simulink library "sixDoFDynamicsCoupled"  (R2020a)
settings: Solver=VariableStepAuto  StartTime=0.0  StopTime=10.0  RelTol=1e-3
undefined symbols (not defined in the file): initPos, vcl
libraries: vrlib x7, eulAng2RotMat_ul x1, eulDot x1
settings Model: Creator=jldanie5  LastModifiedBy=Ayaz
settings DataIOCC: ReturnWorkspaceOutputs=off
settings DebuggingCC: ArithmeticOperatorsInVariantConditions=warning
settings SFSimCC: CustomCodeUndefinedFunction=UseInterfaceOnly

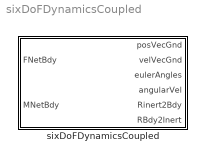
== system sixDoFDynamicsCoupled ==
  sixDoFDynamicsCoupled : Subsystem  VariantControl=(default)  mask{massMatrix=vcl.M6x6.Value, addedMassMatrix=vcl.Ma6x6.Value, rCM_LE=vcl.rCM_B.Value, initPosCM=vcl.initPosVecGnd.Value, initVelCM=vcl.initVelVecBdy.Value, initEulAngs=vcl.initEulAng.Value, initAngVel=vcl.initAngVelVec.Value}
      mask prompts: massMatrix "6x6 Mass Matrix"; addedMassMatrix "6x6 Added Mass Matrix"; rCM_LE "Center of mass position vec wrt leading edge in body frame"; initPosCM "Initial position"; initVelCM "Initial velocity"; initEulAngs "Initial Euler Angles"; initAngVel "Initial Angular Velocity Vec"
      mask init:
      | Mnet = massMatrix - addedMassMatrix;
      | invMnet = inv(Mnet);
      | mAddedTimesMInvMinusEye = addedMassMatrix*inv(massMatrix) - eye(6);
      | 
      | % mass
      | m = massMatrix(1,1);
      | % inertia about body frame origin
      | J = massMatrix(4:6,4:6);
      | % initial velocity of body frame origin
      | initVelB = initVelCM - cross(initAngVel,rCM_LE);
      mask DialogControl Container6 Prompt: Mass Matrices
      mask DialogControl Container4 Prompt: Point Locations
      mask DialogControl Container3 Prompt: Initial Conditions

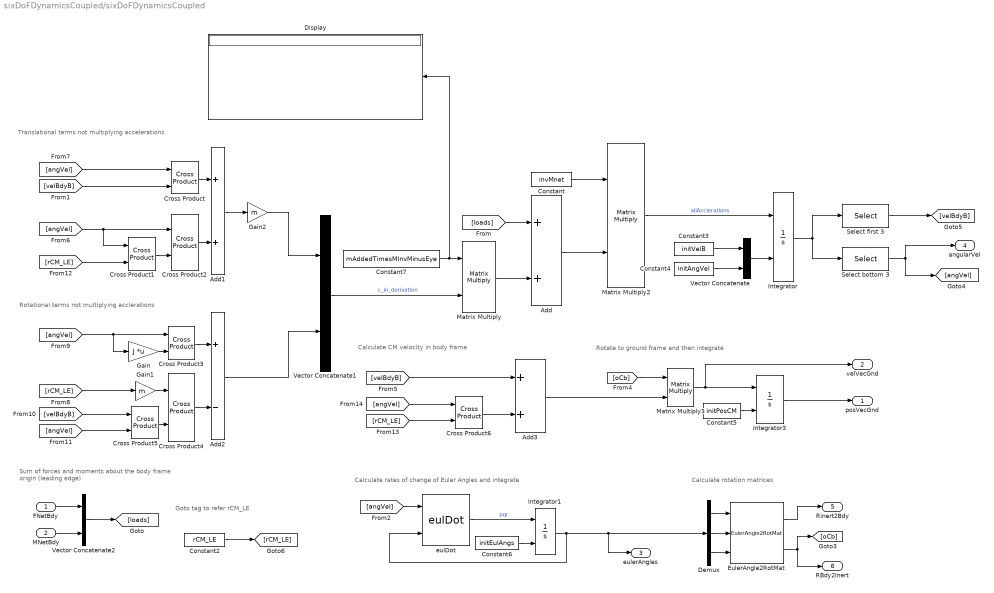
== system sixDoFDynamicsCoupled/sixDoFDynamicsCoupled ==
  note: Calculate rotation matrices
  note: Calculate CM velocity in body frame
  note: Goto tag to refer rCM_LE
  note: Rotational terms not multiplying acclerations
  note: Translational terms not multiplying accelerations
  note: Sum of forces and moments about the
      | body frame origin (leading edge)
  note: Rotate to ground frame and then integrate
  note: Calculate rates of change of Euler Angles and integrate
  FNetBdy : Inport
  MNetBdy : Inport  Port=2
  Add : Sum
  Add1 : Sum
  Add2 : Sum  Inputs=+-
  Add3 : Sum
  Constant : Constant  Value=invMnet  VectorParams1D=off
  Constant2 : Constant  Value=rCM_LE  VectorParams1D=off
  Constant3 : Constant  Value=initVelB  VectorParams1D=off
  Constant4 : Constant  Value=initAngVel  VectorParams1D=off
  Constant5 : Constant  Value=initPosCM  VectorParams1D=off
  Constant6 : Constant  Value=initEulAngs  VectorParams1D=off
  Constant7 : Constant  Value=mAddedTimesMInvMinusEye  VectorParams1D=off
  Cross Product{,1..6} (7 alike) : vrlib/Utilities/Cross Product
  Demux : Demux  Outputs=3
  Display : Display
  EulerAngle2RotMat : eulAng2RotMat_ul/EulerAngle2RotMat  SystemSampleTime=-1  Latency=0  AutoFrameSizeCalculation=off
  Gain : Gain  Gain=J  Multiplication=Matrix(K*u)
  Gain1 : Gain  Gain=m
  Gain2 : Gain  Gain=m
  Integrator : Integrator  InitialConditionSource=external
  Integrator1 : Integrator  InitialConditionSource=external  InitialCondition=initEulAngs
  Integrator3 : Integrator  InitialConditionSource=external  InitialCondition=initPos
  Matrix Multiply : Product  Multiplication=Matrix(*)
  Matrix Multiply2 : Product  Multiplication=Matrix(*)
  Matrix Multiply3 : Product  Multiplication=Matrix(*)
  Select bottom 3 : Selector  NumberOfDimensions=2  InputPortWidth=6  IndexOptions=Index vector (dialog),Index vector (dialog)  Indices=[4 5 6],1  OutputSizes=1,1
  Select first 3 : Selector  NumberOfDimensions=2  InputPortWidth=6  IndexOptions=Index vector (dialog),Index vector (dialog)  Indices=[1 2 3],1  OutputSizes=1,1
  Vector Concatenate : Concatenate
  Vector Concatenate1 : Concatenate
  Vector Concatenate2 : Concatenate
  eulDot : eulDot/eulDot  SystemSampleTime=-1  Latency=0  AutoFrameSizeCalculation=off
  posVecGnd : Outport  VectorParamsAs1DForOutWhenUnconnected=off
  velVecGnd : Outport  Port=2  VectorParamsAs1DForOutWhenUnconnected=off
  eulerAngles : Outport  Port=3  VectorParamsAs1DForOutWhenUnconnected=off
  angularVel : Outport  Port=4  VectorParamsAs1DForOutWhenUnconnected=off
  Rinert2Bdy : Outport  Port=5  VectorParamsAs1DForOutWhenUnconnected=off
  RBdy2Inert : Outport  Port=6  VectorParamsAs1DForOutWhenUnconnected=off
  wires:
  Vector Concatenate2/1 -> [loads]
  Constant/1 -> Matrix Multiply2/1
  Matrix Multiply2/1 -> Integrator/1  "allAcclerations"
  Constant4/1 -> Vector Concatenate/2
  Vector Concatenate/1 -> Integrator/2
  Demux/3 -> EulerAngle2RotMat/3
  Demux/1 -> EulerAngle2RotMat/1
  EulerAngle2RotMat/2 -> RBdy2Inert/1, [oCb]
  Integrator3/1 -> posVecGnd/1
  Demux/2 -> EulerAngle2RotMat/2
  Constant5/1 -> Integrator3/2
  Integrator1/1 -> eulerAngles/1, Demux/1, eulDot/2
  eulDot/1 -> Integrator1/1  "pqr"
  Constant6/1 -> Integrator1/2
  Matrix Multiply3/1 -> Integrator3/1, velVecGnd/1
  EulerAngle2RotMat/1 -> Rinert2Bdy/1
  Constant3/1 -> Vector Concatenate/1
  Select first 3/1 -> [velBdyB]
  [oCb] -> Matrix Multiply3/1
  [angVel] -> Cross Product3/1, Gain/1
  Gain/1 -> Cross Product3/2
  [rCM_LE] -> Gain1/1
  Gain1/1 -> Cross Product4/1
  [velBdyB] -> Cross Product5/1
  [angVel] -> Cross Product5/2
  Cross Product5/1 -> Cross Product4/2
  Cross Product3/1 -> Add2/1
  Cross Product4/1 -> Add2/2
  Add2/1 -> Vector Concatenate1/2
  FNetBdy/1 -> Vector Concatenate2/1
  MNetBdy/1 -> Vector Concatenate2/2
  Add1/1 -> Gain2/1
  Constant2/1 -> [rCM_LE]
  Cross Product/1 -> Add1/1
  Cross Product1/1 -> Cross Product2/2
  [velBdyB] -> Cross Product/2
  Cross Product2/1 -> Add1/2
  [angVel] -> Cross Product/1
  [angVel] -> Cross Product1/1, Cross Product2/1
  Gain2/1 -> Vector Concatenate1/1
  Vector Concatenate1/1 -> Matrix Multiply/2  "c_in_derivation"
  Constant7/1 -> Display/1, Matrix Multiply/1
  Matrix Multiply/1 -> Add/2
  [loads] -> Add/1
  Add/1 -> Matrix Multiply2/2
  Integrator/1 -> Select bottom 3/1, Select first 3/1
  Select bottom 3/1 -> [angVel], angularVel/1
  [rCM_LE] -> Cross Product1/2
  [rCM_LE] -> Cross Product6/2
  [angVel] -> Cross Product6/1
  [velBdyB] -> Add3/1
  Cross Product6/1 -> Add3/2
  Add3/1 -> Matrix Multiply3/2
  [angVel] -> eulDot/1
